simulink model "MHILSimHWImpl"  (R2024a)
settings: Solver=FixedStepDiscrete  StartTime=0.0  StopTime=2e-4  FixedStep=4e-9  RelTol=1e-3
values from neighbouring files (symbols this model uses):
  cfg = tddbl_model    [HILSimModel.m]
undefined symbols (not defined in the file or in its folder): AXI4, dt, hw, ip, Lite, xc7z020clg400
libraries: hdlBasic x1497, hdlUtilities x3, vmcUtilities x1
(part 5 of 11)

== system MHILSimHWImpl/hilsim_ipcore/proc_domain/sel_addrs_slice_2 ==
  Bus Creator : BusCreator  Inputs=6
  Constant : hdlBasic/Constant  const=ip.nlfaddr.slice2_u0  gui_display_data_type=Fixed-point  arith_type=Unsigned  n_bits=8  bin_pt=0  preci_type=Single  exp_width=8  frac_width=24  explicit_period=off  period=1  XmcBlockStatus=1  maskContainerNames=tabcontainer1  block_type=constant  block_config=sysgen:Constant_config
  Constant1 : hdlBasic/Constant  const=ip.nlfaddr.slice2_u1  gui_display_data_type=Fixed-point  arith_type=Unsigned  n_bits=8  bin_pt=0  preci_type=Single  exp_width=8  frac_width=24  explicit_period=off  period=1  XmcBlockStatus=1  maskContainerNames=tabcontainer1  block_type=constant  block_config=sysgen:Constant_config
  Constant2 : hdlBasic/Constant  const=ip.nlfaddr.slice2_x0  gui_display_data_type=Fixed-point  arith_type=Unsigned  n_bits=8  bin_pt=0  preci_type=Single  exp_width=8  frac_width=24  explicit_period=off  period=1  XmcBlockStatus=1  maskContainerNames=tabcontainer1  block_type=constant  block_config=sysgen:Constant_config
  Constant3 : hdlBasic/Constant  const=ip.nlfaddr.slice2_x1  gui_display_data_type=Fixed-point  arith_type=Unsigned  n_bits=8  bin_pt=0  preci_type=Single  exp_width=8  frac_width=24  explicit_period=off  period=1  XmcBlockStatus=1  maskContainerNames=tabcontainer1  block_type=constant  block_config=sysgen:Constant_config
  Constant4 : hdlBasic/Constant  const=ip.nlfaddr.slice2_xd0  gui_display_data_type=Fixed-point  arith_type=Unsigned  n_bits=8  bin_pt=0  preci_type=Single  exp_width=8  frac_width=24  explicit_period=off  period=1  XmcBlockStatus=1  maskContainerNames=tabcontainer1  block_type=constant  block_config=sysgen:Constant_config
  Constant5 : hdlBasic/Constant  const=ip.nlfaddr.slice2_xd1  gui_display_data_type=Fixed-point  arith_type=Unsigned  n_bits=8  bin_pt=0  preci_type=Single  exp_width=8  frac_width=24  explicit_period=off  period=1  XmcBlockStatus=1  maskContainerNames=tabcontainer1  block_type=constant  block_config=sysgen:Constant_config
  nlf_sel_addrs : Outport
  wires:
  Bus Creator/1 -> nlf_sel_addrs/1
  Constant/1 -> Bus Creator/1  "sel_u0"
  Constant1/1 -> Bus Creator/2  "sel_u1"
  Constant2/1 -> Bus Creator/3  "sel_x0"
  Constant3/1 -> Bus Creator/4  "sel_x1"
  Constant4/1 -> Bus Creator/5  "sel_xd0"
  Constant5/1 -> Bus Creator/6  "sel_xd1"

== system MHILSimHWImpl/hilsim_ipcore/proc_domain/slice_0 ==
  note: clk=3
  note: clk=6 (linear)
      | clk=18 (nonlinear)
  note: FB: max_clk=32
  note: clk=3
  note: clk=5
  note: clk=5
  u : Inport
  nlf_cfg_bus : Inport  Port=2
  slice_cfg : Inport  Port=3
  nlf_switch_bus : Inport  Port=4
  nlf_sel_addrs : Inport  Port=5
  reset_in : Inport  Port=6
  Bus Selector : BusSelector  OutputSignals=signal1,signal2,signal3,signal4,signal5,signal6,signal7,signal8,signal9,signal10,signal11,signal12,signal13,signal14,signal15,signal16
  Register{1..10,12} (11 alike) : hdlBasic/Register  init=0  rst=off  en=off  XmcBlockStatus=1  maskContainerNames=tabcontainer1  block_type=register  block_config=sysgen:Register_config
  fb_func : Subsystem
  fb_resync : Subsystem
  int_xddot_xdot : Subsystem
  int_xdot_x : Subsystem
  sample_sync : hdlUtilities/Clock Enable Probe  inherit_constraints=on  XmcBlockStatus=1  maskContainerNames=group1  block_type=ceprobe  block_config=sysgen:CEProbe_config
  u_downsample : hdlBasic/Down Sample  sample_ratio=hw.oversample  sample_phase=First Value of Frame  en=off  rst=off  latency=0  XmcBlockStatus=1  maskContainerNames=group1  block_type=dsamp  block_config=sysgen:Downsample_config
  u_upsample : hdlBasic/Up Sample  sample_ratio=hw.oversample  copy_samples=on  en=off  latency=1  XmcBlockStatus=1  maskContainerNames=group1  block_type=usamp  block_config=sysgen:Upsample_config
  x_psc : Subsystem
  xdot_psc : Subsystem
  x_sync : Outport
  xd_sync : Outport  Port=2
  xdd_sync : Outport  Port=3
  wires:
  x_psc/1(out) -> fb_resync/4(x)
  xdot_psc/1(out) -> fb_resync/5(xd), int_xdot_x/3(xdot)
  fb_func/1(xdd) -> int_xddot_xdot/3(xdot), fb_resync/6(xdd)
  sample_sync/1 -> fb_resync/1(ts_sync_in), int_xddot_xdot/1(ts_sync_in), int_xdot_x/1(ts_sync_in)
  nlf_cfg_bus/1 -> fb_func/4(nlf_cfg_bus)
  int_xdot_x/1(x) -> x_psc/1(in)
  u_downsample/1 -> sample_sync/1, u_upsample/1
  fb_resync/1(u_sync) -> fb_func/1(u)
  Bus Selector/1 -> fb_func/7(x_mux)  "<signal1>"
  Bus Selector/2 -> Register4/1  "<signal2>"
  Bus Selector/3 -> fb_func/9(x_nlf_presc)  "<signal3>"
  Bus Selector/4 -> fb_func/10(x_nlf_gain)  "<signal4>"
  Bus Selector/5 -> fb_func/11(xd_mux)  "<signal5>"
  Bus Selector/6 -> Register5/1  "<signal6>"
  Bus Selector/7 -> fb_func/13(xd_nlf_presc)  "<signal7>"
  Bus Selector/8 -> fb_func/14(xd_nlf_gain)  "<signal8>"
  Bus Selector/9 -> fb_func/15(u_mux)  "<signal9>"
  Bus Selector/10 -> Register6/1  "<signal10>"
  Bus Selector/11 -> fb_func/17(u_nlf_presc)  "<signal11>"
  Bus Selector/12 -> fb_func/18(u_nlf_gain)  "<signal12>"
  slice_cfg/1 -> Bus Selector/1
  int_xddot_xdot/1(x) -> xdot_psc/1(in)
  Bus Selector/13 -> Register12/1  "<signal13>"
  Bus Selector/14 -> Register1/1  "<signal14>"
  Bus Selector/15 -> Register2/1  "<signal15>"
  Bus Selector/16 -> Register3/1  "<signal16>"
  u_upsample/1 -> fb_resync/3(u)
  fb_resync/2(x_sync) -> x_sync/1, fb_func/2(x)
  fb_resync/3(xd_sync) -> xd_sync/1, fb_func/3(xd)
  u/1 -> u_downsample/1
  Register12/1 -> Register8/1
  Register1/1 -> Register7/1
  Register2/1 -> Register9/1
  Register3/1 -> Register10/1
  Register4/1 -> fb_func/8(x_gain)
  Register5/1 -> fb_func/12(xd_gain)
  Register6/1 -> fb_func/16(u_gain)
  reset_in/1 -> fb_resync/2(reset_in), int_xdot_x/2(reset_in), int_xddot_xdot/2(reset_in)
  Register8/1 -> xdot_psc/2(presc_shift)
  Register7/1 -> xdot_psc/3(presc_mul)
  Register10/1 -> x_psc/3(presc_mul)
  Register9/1 -> x_psc/2(presc_shift)
  fb_resync/4(xdd_sync) -> xdd_sync/1
  nlf_switch_bus/1 -> fb_func/5(nlf_switch_bus)
  nlf_sel_addrs/1 -> fb_func/6(nlf_sel_addrs)

== system MHILSimHWImpl/hilsim_ipcore/proc_domain/slice_1 ==
  note: clk=3
  note: clk=6 (linear)
      | clk=18 (nonlinear)
  note: FB: max_clk=32
  note: clk=3
  note: clk=5
  note: clk=5
  u : Inport
  nlf_cfg_bus : Inport  Port=2
  slice_cfg : Inport  Port=3
  nlf_switch_bus : Inport  Port=4
  nlf_sel_addrs : Inport  Port=5
  reset_in : Inport  Port=6
  Bus Selector : BusSelector  OutputSignals=signal1,signal2,signal3,signal4,signal5,signal6,signal7,signal8,signal9,signal10,signal11,signal12,signal13,signal14,signal15,signal16
  Register{1..10,12} (11 alike) : hdlBasic/Register  init=0  rst=off  en=off  XmcBlockStatus=1  maskContainerNames=tabcontainer1  block_type=register  block_config=sysgen:Register_config
  fb_func : Subsystem
  fb_resync : Subsystem
  int_xddot_xdot : Subsystem
  int_xdot_x : Subsystem
  sample_sync : hdlUtilities/Clock Enable Probe  inherit_constraints=on  XmcBlockStatus=1  maskContainerNames=group1  block_type=ceprobe  block_config=sysgen:CEProbe_config
  u_downsample : hdlBasic/Down Sample  sample_ratio=hw.oversample  sample_phase=First Value of Frame  en=off  rst=off  latency=0  XmcBlockStatus=1  maskContainerNames=group1  block_type=dsamp  block_config=sysgen:Downsample_config
  u_upsample : hdlBasic/Up Sample  sample_ratio=hw.oversample  copy_samples=on  en=off  latency=1  XmcBlockStatus=1  maskContainerNames=group1  block_type=usamp  block_config=sysgen:Upsample_config
  x_psc : Subsystem
  xdot_psc : Subsystem
  x_sync : Outport
  xd_sync : Outport  Port=2
  xdd_sync : Outport  Port=3
  wires:
  x_psc/1(out) -> fb_resync/4(x)
  xdot_psc/1(out) -> fb_resync/5(xd), int_xdot_x/3(xdot)
  fb_func/1(xdd) -> int_xddot_xdot/3(xdot), fb_resync/6(xdd)
  sample_sync/1 -> fb_resync/1(ts_sync_in), int_xddot_xdot/1(ts_sync_in), int_xdot_x/1(ts_sync_in)
  nlf_cfg_bus/1 -> fb_func/4(nlf_cfg_bus)
  int_xdot_x/1(x) -> x_psc/1(in)
  u_downsample/1 -> sample_sync/1, u_upsample/1
  fb_resync/1(u_sync) -> fb_func/1(u)
  Bus Selector/1 -> fb_func/7(x_mux)  "<signal1>"
  Bus Selector/2 -> Register4/1  "<signal2>"
  Bus Selector/3 -> fb_func/9(x_nlf_presc)  "<signal3>"
  Bus Selector/4 -> fb_func/10(x_nlf_gain)  "<signal4>"
  Bus Selector/5 -> fb_func/11(xd_mux)  "<signal5>"
  Bus Selector/6 -> Register5/1  "<signal6>"
  Bus Selector/7 -> fb_func/13(xd_nlf_presc)  "<signal7>"
  Bus Selector/8 -> fb_func/14(xd_nlf_gain)  "<signal8>"
  Bus Selector/9 -> fb_func/15(u_mux)  "<signal9>"
  Bus Selector/10 -> Register6/1  "<signal10>"
  Bus Selector/11 -> fb_func/17(u_nlf_presc)  "<signal11>"
  Bus Selector/12 -> fb_func/18(u_nlf_gain)  "<signal12>"
  slice_cfg/1 -> Bus Selector/1
  int_xddot_xdot/1(x) -> xdot_psc/1(in)
  Bus Selector/13 -> Register12/1  "<signal13>"
  Bus Selector/14 -> Register1/1  "<signal14>"
  Bus Selector/15 -> Register2/1  "<signal15>"
  Bus Selector/16 -> Register3/1  "<signal16>"
  u_upsample/1 -> fb_resync/3(u)
  fb_resync/2(x_sync) -> x_sync/1, fb_func/2(x)
  fb_resync/3(xd_sync) -> xd_sync/1, fb_func/3(xd)
  u/1 -> u_downsample/1
  Register12/1 -> Register8/1
  Register1/1 -> Register7/1
  Register2/1 -> Register9/1
  Register3/1 -> Register10/1
  Register4/1 -> fb_func/8(x_gain)
  Register5/1 -> fb_func/12(xd_gain)
  Register6/1 -> fb_func/16(u_gain)
  reset_in/1 -> fb_resync/2(reset_in), int_xdot_x/2(reset_in), int_xddot_xdot/2(reset_in)
  Register8/1 -> xdot_psc/2(presc_shift)
  Register7/1 -> xdot_psc/3(presc_mul)
  Register10/1 -> x_psc/3(presc_mul)
  Register9/1 -> x_psc/2(presc_shift)
  fb_resync/4(xdd_sync) -> xdd_sync/1
  nlf_switch_bus/1 -> fb_func/5(nlf_switch_bus)
  nlf_sel_addrs/1 -> fb_func/6(nlf_sel_addrs)

== system MHILSimHWImpl/hilsim_ipcore/proc_domain/slice_2 ==
  note: clk=3
  note: clk=6 (linear)
      | clk=18 (nonlinear)
  note: FB: max_clk=32
  note: clk=3
  note: clk=5
  note: clk=5
  u : Inport
  nlf_cfg_bus : Inport  Port=2
  slice_cfg : Inport  Port=3
  nlf_switch_bus : Inport  Port=4
  nlf_sel_addrs : Inport  Port=5
  reset_in : Inport  Port=6
  Bus Selector : BusSelector  OutputSignals=signal1,signal2,signal3,signal4,signal5,signal6,signal7,signal8,signal9,signal10,signal11,signal12,signal13,signal14,signal15,signal16
  Register{1..10,12} (11 alike) : hdlBasic/Register  init=0  rst=off  en=off  XmcBlockStatus=1  maskContainerNames=tabcontainer1  block_type=register  block_config=sysgen:Register_config
  fb_func : Subsystem
  fb_resync : Subsystem
  int_xddot_xdot : Subsystem
  int_xdot_x : Subsystem
  sample_sync : hdlUtilities/Clock Enable Probe  inherit_constraints=on  XmcBlockStatus=1  maskContainerNames=group1  block_type=ceprobe  block_config=sysgen:CEProbe_config
  u_downsample : hdlBasic/Down Sample  sample_ratio=hw.oversample  sample_phase=First Value of Frame  en=off  rst=off  latency=0  XmcBlockStatus=1  maskContainerNames=group1  block_type=dsamp  block_config=sysgen:Downsample_config
  u_upsample : hdlBasic/Up Sample  sample_ratio=hw.oversample  copy_samples=on  en=off  latency=1  XmcBlockStatus=1  maskContainerNames=group1  block_type=usamp  block_config=sysgen:Upsample_config
  x_psc : Subsystem
  xdot_psc : Subsystem
  x_sync : Outport
  xd_sync : Outport  Port=2
  xdd_sync : Outport  Port=3
  wires:
  x_psc/1(out) -> fb_resync/4(x)
  xdot_psc/1(out) -> fb_resync/5(xd), int_xdot_x/3(xdot)
  fb_func/1(xdd) -> int_xddot_xdot/3(xdot), fb_resync/6(xdd)
  sample_sync/1 -> fb_resync/1(ts_sync_in), int_xddot_xdot/1(ts_sync_in), int_xdot_x/1(ts_sync_in)
  nlf_cfg_bus/1 -> fb_func/4(nlf_cfg_bus)
  int_xdot_x/1(x) -> x_psc/1(in)
  u_downsample/1 -> sample_sync/1, u_upsample/1
  fb_resync/1(u_sync) -> fb_func/1(u)
  Bus Selector/1 -> fb_func/7(x_mux)  "<signal1>"
  Bus Selector/2 -> Register4/1  "<signal2>"
  Bus Selector/3 -> fb_func/9(x_nlf_presc)  "<signal3>"
  Bus Selector/4 -> fb_func/10(x_nlf_gain)  "<signal4>"
  Bus Selector/5 -> fb_func/11(xd_mux)  "<signal5>"
  Bus Selector/6 -> Register5/1  "<signal6>"
  Bus Selector/7 -> fb_func/13(xd_nlf_presc)  "<signal7>"
  Bus Selector/8 -> fb_func/14(xd_nlf_gain)  "<signal8>"
  Bus Selector/9 -> fb_func/15(u_mux)  "<signal9>"
  Bus Selector/10 -> Register6/1  "<signal10>"
  Bus Selector/11 -> fb_func/17(u_nlf_presc)  "<signal11>"
  Bus Selector/12 -> fb_func/18(u_nlf_gain)  "<signal12>"
  slice_cfg/1 -> Bus Selector/1
  int_xddot_xdot/1(x) -> xdot_psc/1(in)
  Bus Selector/13 -> Register12/1  "<signal13>"
  Bus Selector/14 -> Register1/1  "<signal14>"
  Bus Selector/15 -> Register2/1  "<signal15>"
  Bus Selector/16 -> Register3/1  "<signal16>"
  u_upsample/1 -> fb_resync/3(u)
  fb_resync/2(x_sync) -> x_sync/1, fb_func/2(x)
  fb_resync/3(xd_sync) -> xd_sync/1, fb_func/3(xd)
  u/1 -> u_downsample/1
  Register12/1 -> Register8/1
  Register1/1 -> Register7/1
  Register2/1 -> Register9/1
  Register3/1 -> Register10/1
  Register4/1 -> fb_func/8(x_gain)
  Register5/1 -> fb_func/12(xd_gain)
  Register6/1 -> fb_func/16(u_gain)
  reset_in/1 -> fb_resync/2(reset_in), int_xdot_x/2(reset_in), int_xddot_xdot/2(reset_in)
  Register8/1 -> xdot_psc/2(presc_shift)
  Register7/1 -> xdot_psc/3(presc_mul)
  Register10/1 -> x_psc/3(presc_mul)
  Register9/1 -> x_psc/2(presc_shift)
  fb_resync/4(xdd_sync) -> xdd_sync/1
  nlf_switch_bus/1 -> fb_func/5(nlf_switch_bus)
  nlf_sel_addrs/1 -> fb_func/6(nlf_sel_addrs)

== system MHILSimHWImpl/hilsim_ipcore/proc_domain/adc_nlf/nlf_adc0 ==
  note: Signal should now be normalized
      | to range -1 to 1.
  x : Inport
  presc : Inport  Port=2
  gain : Inport  Port=3
  cfg_select : Inport  Port=4
  cfg_addr : Inport  Port=5
  cfg_data : Inport  Port=6
  cfg_we : Inport  Port=7
  AddSub : hdlBasic/AddSub  mode=Addition  use_carryin=off  use_carryout=off  en=off  latency=1  precision=User Defined  arith_type=Unsigned  n_bits=ip.f_nlf.lut_addr_bits  bin_pt=0  quantization=Truncate  overflow=Wrap  use_behavioral_HDL=off  hw_selection=Fabric  pipelined=off  XmcBlockStatus=1  maskContainerNames=tabcontainer1  block_type=addsub  block_config=sysgen:Addsub_config
  AddSub1 : hdlBasic/AddSub  mode=Subtraction  use_carryin=off  use_carryout=off  en=off  latency=2  precision=User Defined  arith_type="Signed  (2's comp)"  n_bits=dt.slice.sz  bin_pt=dt.slice.bin  quantization=Truncate  overflow=Wrap  use_behavioral_HDL=off  hw_selection=Fabric  pipelined=off  XmcBlockStatus=1  maskContainerNames=tabcontainer1  block_type=addsub  block_config=sysgen:Addsub_config
  LUT : hdlBasic/Dual Port RAM  depth=ip.f_nlf.lut_sz  initVector=cfg.adc0_nlf.lut  distributed_mem=Block RAM  init_a=0  init_b=0  rst_a=off  rst_b=off  en_a=off  en_b=off  latency=1  write_mode_A=Read After Write  write_mode_B=Read After Write  explicit_period=[]  period=[]  simulation_type=fast_sim  XmcBlockStatus=1  maskContainerNames=tabcontainer1  block_type=dpram  block_config=sysgen:Dpram_config  optimize=Area
      settings: infoedit=[]
  Reinterpret : hdlBasic/Reinterpret  force_arith_type=on  arith_type=Unsigned  force_bin_pt=on  bin_pt=0  XmcBlockStatus=1  maskContainerNames=group1  block_type=reinterpret  block_config=sysgen:Reinterpret_config
  add_interpolate : hdlBasic/AddSub  mode=Addition  use_carryin=off  use_carryout=off  en=off  latency=1  precision=User Defined  arith_type="Signed  (2's comp)"  n_bits=dt.slice.sz  bin_pt=dt.slice.bin  quantization=Truncate  overflow=Wrap  use_behavioral_HDL=off  hw_selection=Fabric  pipelined=off  XmcBlockStatus=1  maskContainerNames=tabcontainer1  block_type=addsub  block_config=sysgen:Addsub_config
  addra_mux : hdlBasic/Mux  inputs=2  en=off  latency=1  precision=Full  arith_type=Unsigned  n_bits=16  bin_pt=14  quantization=Truncate  overflow=Wrap  XmcBlockStatus=1  maskContainerNames=tabcontainer1  block_type=mux  block_config=sysgen:Mux_config
  bool_zero_we : hdlBasic/Constant  const=0  gui_display_data_type=Boolean  arith_type=Boolean  n_bits=16  bin_pt=14  preci_type=Single  exp_width=8  frac_width=24  explicit_period=off  period=1  XmcBlockStatus=1  maskContainerNames=tabcontainer1  block_type=constant  block_config=sysgen:Constant_config
  bool_zero_wea : hdlBasic/Constant  const=0  gui_display_data_type=Boolean  arith_type=Boolean  n_bits=16  bin_pt=14  preci_type=Single  exp_width=8  frac_width=24  explicit_period=off  period=1  XmcBlockStatus=1  maskContainerNames=tabcontainer1  block_type=constant  block_config=sysgen:Constant_config
  cast_cutoff_lsbits : hdlBasic/Convert  gui_display_data_type=Fixed-point  arith_type="Signed  (2's comp)"  n_bits=ip.f_nlf.lut_addr_bits  bin_pt=ip.f_nlf.lut_addr_bits-1  float_type=Single  exp_bits=8  fraction_bits=24  quantization=Truncate  overflow=Wrap  en=off  latency=0  pipeline=off  XmcBlockStatus=1  maskContainerNames=group2  block_type=convert  block_config=sysgen:Convert_config  block_width=595  block_height=885
  cast_to_dt/slice : hdlBasic/Convert  gui_display_data_type=Fixed-point  arith_type="Signed  (2's comp)"  n_bits=dt.slice.sz  bin_pt=dt.slice.bin  float_type=Single  exp_bits=8  fraction_bits=24  quantization=Truncate  overflow=Wrap  en=off  latency=0  pipeline=off  XmcBlockStatus=1  maskContainerNames=group2  block_type=convert  block_config=sysgen:Convert_config  block_width=595  block_height=885
  const_1 : hdlBasic/Constant  const=1.0  gui_display_data_type=Fixed-point  arith_type=Unsigned  n_bits=ip.f_nlf.lut_addr_bits  bin_pt=0  preci_type=Single  exp_width=8  frac_width=24  explicit_period=off  period=1  XmcBlockStatus=1  maskContainerNames=tabcontainer1  block_type=constant  block_config=sysgen:Constant_config
  const_1_interp : hdlBasic/Constant  const=1  gui_display_data_type=Fixed-point  arith_type=Signed (2's comp)  n_bits=dt.slice.sz  bin_pt=dt.slice.bin  preci_type=Single  exp_width=8  frac_width=24  explicit_period=off  period=1  XmcBlockStatus=1  maskContainerNames=tabcontainer1  block_type=constant  block_config=sysgen:Constant_config
  cutoff_msbits : hdlBasic/Slice  nbits=dt.slice.sz - ip.f_nlf.lut_addr_bits-1  boolean_output=off  mode=Lower Bit Location + Width  bit1=0  base1=MSB of Input  bit0=0  base0=LSB of Input  XmcBlockStatus=1  maskContainerNames=group1  block_type=slice  block_config=sysgen:Slice_config
  delay_sync_interpolate : hdlBasic/Delay  rst=off  en=off  latency=2  reg_retiming=off  XmcBlockStatus=1  maskContainerNames=group1  block_type=delay  block_config=sysgen:Delay_config
  dina_mux : hdlBasic/Mux  inputs=2  en=off  latency=1  precision=Full  arith_type=Unsigned  n_bits=16  bin_pt=14  quantization=Truncate  overflow=Wrap  XmcBlockStatus=1  maskContainerNames=tabcontainer1  block_type=mux  block_config=sysgen:Mux_config
  mult_a : hdlBasic/Mult  precision=User Defined  arith_type="Signed  (2's comp)"  n_bits=dt.slice.sz  bin_pt=dt.slice.bin  quantization=Truncate  overflow=Wrap  en=off  latency=3  opt_float=off  fp_mult_usage=No Usage  use_behavioral_HDL=off  opt=Speed  use_embedded=on  optimum_pipeline=off  pipeline=on  use_rpm=on  placement_style=Triangular  XmcBlockStatus=1  maskContainerNames=group1  block_type=mult  block_config=sysgen:Mult_config  block_width=598  block_height=876
  mult_b : hdlBasic/Mult  precision=User Defined  arith_type="Signed  (2's comp)"  n_bits=dt.slice.sz  bin_pt=dt.slice.bin  quantization=Truncate  overflow=Wrap  en=off  latency=3  opt_float=off  fp_mult_usage=No Usage  use_behavioral_HDL=off  opt=Speed  use_embedded=on  optimum_pipeline=off  pipeline=on  use_rpm=on  placement_style=Triangular  XmcBlockStatus=1  maskContainerNames=group1  block_type=mult  block_config=sysgen:Mult_config  block_width=598  block_height=876
  mult_inp_scale : hdlBasic/Mult  precision=User Defined  arith_type="Signed  (2's comp)"  n_bits=dt.slice.sz  bin_pt=dt.slice.sz - 2  quantization=Truncate  overflow=Wrap  en=off  latency=3  opt_float=off  fp_mult_usage=No Usage  use_behavioral_HDL=off  opt=Speed  use_embedded=on  optimum_pipeline=off  pipeline=on  use_rpm=on  placement_style=Triangular  XmcBlockStatus=1  maskContainerNames=group1  block_type=mult  block_config=sysgen:Mult_config  block_width=598  block_height=876
  mult_out_scale : hdlBasic/Mult  precision=User Defined  arith_type="Signed  (2's comp)"  n_bits=dt.slice.sz  bin_pt=dt.slice.bin  quantization=Truncate  overflow=Wrap  en=off  latency=3  opt_float=off  fp_mult_usage=No Usage  use_behavioral_HDL=off  opt=Speed  use_embedded=on  optimum_pipeline=off  pipeline=on  use_rpm=on  placement_style=Triangular  XmcBlockStatus=1  maskContainerNames=group1  block_type=mult  block_config=sysgen:Mult_config  block_width=598  block_height=876
  reint_sliced : hdlBasic/Reinterpret  force_arith_type=on  arith_type=Unsigned  force_bin_pt=on  bin_pt=dt.slice.sz - ip.f_nlf.lut_addr_bits-1  XmcBlockStatus=1  maskContainerNames=group1  block_type=reinterpret  block_config=sysgen:Reinterpret_config
  wea_mux : hdlBasic/Mux  inputs=2  en=off  latency=1  precision=Full  arith_type=Unsigned  n_bits=16  bin_pt=14  quantization=Truncate  overflow=Wrap  XmcBlockStatus=1  maskContainerNames=tabcontainer1  block_type=mux  block_config=sysgen:Mux_config
  zero_nlf_datatype : hdlBasic/Constant  const=0  gui_display_data_type=Fixed-point  arith_type=Signed (2's comp)  n_bits=dt.nlf.sz  bin_pt=dt.nlf.bin  preci_type=Single  exp_width=8  frac_width=24  explicit_period=off  period=1  XmcBlockStatus=1  maskContainerNames=tabcontainer1  block_type=constant  block_config=sysgen:Constant_config
  zero_nlf_dina : hdlBasic/Constant  const=0  gui_display_data_type=Fixed-point  arith_type=Signed (2's comp)  n_bits=dt.nlf.sz  bin_pt=dt.nlf.bin  preci_type=Single  exp_width=8  frac_width=24  explicit_period=off  period=1  XmcBlockStatus=1  maskContainerNames=tabcontainer1  block_type=constant  block_config=sysgen:Constant_config
  f(x) : Outport
  wires:
  x/1 -> mult_inp_scale/1
  presc/1 -> mult_inp_scale/2
  cast_cutoff_lsbits/1 -> Reinterpret/1
  Reinterpret/1 -> addra_mux/2, AddSub/1
  const_1/1 -> AddSub/2
  AddSub/1 -> LUT/4
  bool_zero_we/1 -> LUT/6
  zero_nlf_datatype/1 -> LUT/5
  LUT/2 -> mult_b/1
  LUT/1 -> mult_a/1
  mult_inp_scale/1 -> cast_cutoff_lsbits/1, cutoff_msbits/1
  cutoff_msbits/1 -> reint_sliced/1
  reint_sliced/1 -> cast_to_dt/slice/1
  cast_to_dt/slice/1 -> AddSub1/2, delay_sync_interpolate/1
  const_1_interp/1 -> AddSub1/1
  delay_sync_interpolate/1 -> mult_b/2
  AddSub1/1 -> mult_a/2
  mult_a/1 -> add_interpolate/1
  mult_b/1 -> add_interpolate/2
  gain/1 -> mult_out_scale/2
  mult_out_scale/1 -> f(x)/1
  dina_mux/1 -> LUT/2
  addra_mux/1 -> LUT/1
  wea_mux/1 -> LUT/3
  bool_zero_wea/1 -> wea_mux/2
  zero_nlf_dina/1 -> dina_mux/2
  cfg_select/1 -> wea_mux/1, dina_mux/1, addra_mux/1
  cfg_addr/1 -> addra_mux/3
  cfg_data/1 -> dina_mux/3
  cfg_we/1 -> wea_mux/3
  add_interpolate/1 -> mult_out_scale/1

== system MHILSimHWImpl/hilsim_ipcore/proc_domain/adc_nlf/nlf_adc1 ==
  note: Signal should now be normalized
      | to range -1 to 1.
  x : Inport
  presc : Inport  Port=2
  gain : Inport  Port=3
  cfg_select : Inport  Port=4
  cfg_addr : Inport  Port=5
  cfg_data : Inport  Port=6
  cfg_we : Inport  Port=7
  AddSub : hdlBasic/AddSub  mode=Addition  use_carryin=off  use_carryout=off  en=off  latency=1  precision=User Defined  arith_type=Unsigned  n_bits=ip.f_nlf.lut_addr_bits  bin_pt=0  quantization=Truncate  overflow=Wrap  use_behavioral_HDL=off  hw_selection=Fabric  pipelined=off  XmcBlockStatus=1  maskContainerNames=tabcontainer1  block_type=addsub  block_config=sysgen:Addsub_config
  AddSub1 : hdlBasic/AddSub  mode=Subtraction  use_carryin=off  use_carryout=off  en=off  latency=2  precision=User Defined  arith_type="Signed  (2's comp)"  n_bits=dt.slice.sz  bin_pt=dt.slice.bin  quantization=Truncate  overflow=Wrap  use_behavioral_HDL=off  hw_selection=Fabric  pipelined=off  XmcBlockStatus=1  maskContainerNames=tabcontainer1  block_type=addsub  block_config=sysgen:Addsub_config
  LUT : hdlBasic/Dual Port RAM  depth=ip.f_nlf.lut_sz  initVector=cfg.adc1_nlf.lut  distributed_mem=Block RAM  init_a=0  init_b=0  rst_a=off  rst_b=off  en_a=off  en_b=off  latency=1  write_mode_A=Read After Write  write_mode_B=Read After Write  explicit_period=[]  period=[]  simulation_type=fast_sim  XmcBlockStatus=1  maskContainerNames=tabcontainer1  block_type=dpram  block_config=sysgen:Dpram_config  optimize=Area
      settings: infoedit=[]
  Reinterpret : hdlBasic/Reinterpret  force_arith_type=on  arith_type=Unsigned  force_bin_pt=on  bin_pt=0  XmcBlockStatus=1  maskContainerNames=group1  block_type=reinterpret  block_config=sysgen:Reinterpret_config
  add_interpolate : hdlBasic/AddSub  mode=Addition  use_carryin=off  use_carryout=off  en=off  latency=1  precision=User Defined  arith_type="Signed  (2's comp)"  n_bits=dt.slice.sz  bin_pt=dt.slice.bin  quantization=Truncate  overflow=Wrap  use_behavioral_HDL=off  hw_selection=Fabric  pipelined=off  XmcBlockStatus=1  maskContainerNames=tabcontainer1  block_type=addsub  block_config=sysgen:Addsub_config
  addra_mux : hdlBasic/Mux  inputs=2  en=off  latency=1  precision=Full  arith_type=Unsigned  n_bits=16  bin_pt=14  quantization=Truncate  overflow=Wrap  XmcBlockStatus=1  maskContainerNames=tabcontainer1  block_type=mux  block_config=sysgen:Mux_config
  bool_zero_we : hdlBasic/Constant  const=0  gui_display_data_type=Boolean  arith_type=Boolean  n_bits=16  bin_pt=14  preci_type=Single  exp_width=8  frac_width=24  explicit_period=off  period=1  XmcBlockStatus=1  maskContainerNames=tabcontainer1  block_type=constant  block_config=sysgen:Constant_config
  bool_zero_wea : hdlBasic/Constant  const=0  gui_display_data_type=Boolean  arith_type=Boolean  n_bits=16  bin_pt=14  preci_type=Single  exp_width=8  frac_width=24  explicit_period=off  period=1  XmcBlockStatus=1  maskContainerNames=tabcontainer1  block_type=constant  block_config=sysgen:Constant_config
  cast_cutoff_lsbits : hdlBasic/Convert  gui_display_data_type=Fixed-point  arith_type="Signed  (2's comp)"  n_bits=ip.f_nlf.lut_addr_bits  bin_pt=ip.f_nlf.lut_addr_bits-1  float_type=Single  exp_bits=8  fraction_bits=24  quantization=Truncate  overflow=Wrap  en=off  latency=0  pipeline=off  XmcBlockStatus=1  maskContainerNames=group2  block_type=convert  block_config=sysgen:Convert_config  block_width=595  block_height=885
  cast_to_dt/slice : hdlBasic/Convert  gui_display_data_type=Fixed-point  arith_type="Signed  (2's comp)"  n_bits=dt.slice.sz  bin_pt=dt.slice.bin  float_type=Single  exp_bits=8  fraction_bits=24  quantization=Truncate  overflow=Wrap  en=off  latency=0  pipeline=off  XmcBlockStatus=1  maskContainerNames=group2  block_type=convert  block_config=sysgen:Convert_config  block_width=595  block_height=885
  const_1 : hdlBasic/Constant  const=1.0  gui_display_data_type=Fixed-point  arith_type=Unsigned  n_bits=ip.f_nlf.lut_addr_bits  bin_pt=0  preci_type=Single  exp_width=8  frac_width=24  explicit_period=off  period=1  XmcBlockStatus=1  maskContainerNames=tabcontainer1  block_type=constant  block_config=sysgen:Constant_config
  const_1_interp : hdlBasic/Constant  const=1  gui_display_data_type=Fixed-point  arith_type=Signed (2's comp)  n_bits=dt.slice.sz  bin_pt=dt.slice.bin  preci_type=Single  exp_width=8  frac_width=24  explicit_period=off  period=1  XmcBlockStatus=1  maskContainerNames=tabcontainer1  block_type=constant  block_config=sysgen:Constant_config
  cutoff_msbits : hdlBasic/Slice  nbits=dt.slice.sz - ip.f_nlf.lut_addr_bits-1  boolean_output=off  mode=Lower Bit Location + Width  bit1=0  base1=MSB of Input  bit0=0  base0=LSB of Input  XmcBlockStatus=1  maskContainerNames=group1  block_type=slice  block_config=sysgen:Slice_config
  delay_sync_interpolate : hdlBasic/Delay  rst=off  en=off  latency=2  reg_retiming=off  XmcBlockStatus=1  maskContainerNames=group1  block_type=delay  block_config=sysgen:Delay_config
  dina_mux : hdlBasic/Mux  inputs=2  en=off  latency=1  precision=Full  arith_type=Unsigned  n_bits=16  bin_pt=14  quantization=Truncate  overflow=Wrap  XmcBlockStatus=1  maskContainerNames=tabcontainer1  block_type=mux  block_config=sysgen:Mux_config
  mult_a : hdlBasic/Mult  precision=User Defined  arith_type="Signed  (2's comp)"  n_bits=dt.slice.sz  bin_pt=dt.slice.bin  quantization=Truncate  overflow=Wrap  en=off  latency=3  opt_float=off  fp_mult_usage=No Usage  use_behavioral_HDL=off  opt=Speed  use_embedded=on  optimum_pipeline=off  pipeline=on  use_rpm=on  placement_style=Triangular  XmcBlockStatus=1  maskContainerNames=group1  block_type=mult  block_config=sysgen:Mult_config  block_width=598  block_height=876
  mult_b : hdlBasic/Mult  precision=User Defined  arith_type="Signed  (2's comp)"  n_bits=dt.slice.sz  bin_pt=dt.slice.bin  quantization=Truncate  overflow=Wrap  en=off  latency=3  opt_float=off  fp_mult_usage=No Usage  use_behavioral_HDL=off  opt=Speed  use_embedded=on  optimum_pipeline=off  pipeline=on  use_rpm=on  placement_style=Triangular  XmcBlockStatus=1  maskContainerNames=group1  block_type=mult  block_config=sysgen:Mult_config  block_width=598  block_height=876
  mult_inp_scale : hdlBasic/Mult  precision=User Defined  arith_type="Signed  (2's comp)"  n_bits=dt.slice.sz  bin_pt=dt.slice.sz - 2  quantization=Truncate  overflow=Wrap  en=off  latency=3  opt_float=off  fp_mult_usage=No Usage  use_behavioral_HDL=off  opt=Speed  use_embedded=on  optimum_pipeline=off  pipeline=on  use_rpm=on  placement_style=Triangular  XmcBlockStatus=1  maskContainerNames=group1  block_type=mult  block_config=sysgen:Mult_config  block_width=598  block_height=876
  mult_out_scale : hdlBasic/Mult  precision=User Defined  arith_type="Signed  (2's comp)"  n_bits=dt.slice.sz  bin_pt=dt.slice.bin  quantization=Truncate  overflow=Wrap  en=off  latency=3  opt_float=off  fp_mult_usage=No Usage  use_behavioral_HDL=off  opt=Speed  use_embedded=on  optimum_pipeline=off  pipeline=on  use_rpm=on  placement_style=Triangular  XmcBlockStatus=1  maskContainerNames=group1  block_type=mult  block_config=sysgen:Mult_config  block_width=598  block_height=876
  reint_sliced : hdlBasic/Reinterpret  force_arith_type=on  arith_type=Unsigned  force_bin_pt=on  bin_pt=dt.slice.sz - ip.f_nlf.lut_addr_bits-1  XmcBlockStatus=1  maskContainerNames=group1  block_type=reinterpret  block_config=sysgen:Reinterpret_config
  wea_mux : hdlBasic/Mux  inputs=2  en=off  latency=1  precision=Full  arith_type=Unsigned  n_bits=16  bin_pt=14  quantization=Truncate  overflow=Wrap  XmcBlockStatus=1  maskContainerNames=tabcontainer1  block_type=mux  block_config=sysgen:Mux_config
  zero_nlf_datatype : hdlBasic/Constant  const=0  gui_display_data_type=Fixed-point  arith_type=Signed (2's comp)  n_bits=dt.nlf.sz  bin_pt=dt.nlf.bin  preci_type=Single  exp_width=8  frac_width=24  explicit_period=off  period=1  XmcBlockStatus=1  maskContainerNames=tabcontainer1  block_type=constant  block_config=sysgen:Constant_config
  zero_nlf_dina : hdlBasic/Constant  const=0  gui_display_data_type=Fixed-point  arith_type=Signed (2's comp)  n_bits=dt.nlf.sz  bin_pt=dt.nlf.bin  preci_type=Single  exp_width=8  frac_width=24  explicit_period=off  period=1  XmcBlockStatus=1  maskContainerNames=tabcontainer1  block_type=constant  block_config=sysgen:Constant_config
  f(x) : Outport
  wires:
  x/1 -> mult_inp_scale/1
  presc/1 -> mult_inp_scale/2
  cast_cutoff_lsbits/1 -> Reinterpret/1
  Reinterpret/1 -> addra_mux/2, AddSub/1
  const_1/1 -> AddSub/2
  AddSub/1 -> LUT/4
  bool_zero_we/1 -> LUT/6
  zero_nlf_datatype/1 -> LUT/5
  LUT/2 -> mult_b/1
  LUT/1 -> mult_a/1
  mult_inp_scale/1 -> cast_cutoff_lsbits/1, cutoff_msbits/1
  cutoff_msbits/1 -> reint_sliced/1
  reint_sliced/1 -> cast_to_dt/slice/1
  cast_to_dt/slice/1 -> AddSub1/2, delay_sync_interpolate/1
  const_1_interp/1 -> AddSub1/1
  delay_sync_interpolate/1 -> mult_b/2
  AddSub1/1 -> mult_a/2
  mult_a/1 -> add_interpolate/1
  mult_b/1 -> add_interpolate/2
  gain/1 -> mult_out_scale/2
  mult_out_scale/1 -> f(x)/1
  dina_mux/1 -> LUT/2
  addra_mux/1 -> LUT/1
  wea_mux/1 -> LUT/3
  bool_zero_wea/1 -> wea_mux/2
  zero_nlf_dina/1 -> dina_mux/2
  cfg_select/1 -> wea_mux/1, dina_mux/1, addra_mux/1
  cfg_addr/1 -> addra_mux/3
  cfg_data/1 -> dina_mux/3
  cfg_we/1 -> wea_mux/3
  add_interpolate/1 -> mult_out_scale/1

== system MHILSimHWImpl/hilsim_ipcore/proc_domain/dac_nlf/nlf_dac0 ==
  note: Signal should now be normalized
      | to range -1 to 1.
  x : Inport
  presc : Inport  Port=2
  gain : Inport  Port=3
  cfg_select : Inport  Port=4
  cfg_addr : Inport  Port=5
  cfg_data : Inport  Port=6
  cfg_we : Inport  Port=7
  AddSub : hdlBasic/AddSub  mode=Addition  use_carryin=off  use_carryout=off  en=off  latency=1  precision=User Defined  arith_type=Unsigned  n_bits=ip.f_nlf.lut_addr_bits  bin_pt=0  quantization=Truncate  overflow=Wrap  use_behavioral_HDL=off  hw_selection=Fabric  pipelined=off  XmcBlockStatus=1  maskContainerNames=tabcontainer1  block_type=addsub  block_config=sysgen:Addsub_config
  AddSub1 : hdlBasic/AddSub  mode=Subtraction  use_carryin=off  use_carryout=off  en=off  latency=2  precision=User Defined  arith_type="Signed  (2's comp)"  n_bits=dt.slice.sz  bin_pt=dt.slice.bin  quantization=Truncate  overflow=Wrap  use_behavioral_HDL=off  hw_selection=Fabric  pipelined=off  XmcBlockStatus=1  maskContainerNames=tabcontainer1  block_type=addsub  block_config=sysgen:Addsub_config
  LUT : hdlBasic/Dual Port RAM  depth=ip.f_nlf.lut_sz  initVector=cfg.dac0_nlf.lut  distributed_mem=Block RAM  init_a=0  init_b=0  rst_a=off  rst_b=off  en_a=off  en_b=off  latency=1  write_mode_A=Read After Write  write_mode_B=Read After Write  explicit_period=[]  period=[]  simulation_type=fast_sim  XmcBlockStatus=1  maskContainerNames=tabcontainer1  block_type=dpram  block_config=sysgen:Dpram_config  optimize=Area
      settings: infoedit=[]
  Reinterpret : hdlBasic/Reinterpret  force_arith_type=on  arith_type=Unsigned  force_bin_pt=on  bin_pt=0  XmcBlockStatus=1  maskContainerNames=group1  block_type=reinterpret  block_config=sysgen:Reinterpret_config
  add_interpolate : hdlBasic/AddSub  mode=Addition  use_carryin=off  use_carryout=off  en=off  latency=1  precision=User Defined  arith_type="Signed  (2's comp)"  n_bits=dt.slice.sz  bin_pt=dt.slice.bin  quantization=Truncate  overflow=Wrap  use_behavioral_HDL=off  hw_selection=Fabric  pipelined=off  XmcBlockStatus=1  maskContainerNames=tabcontainer1  block_type=addsub  block_config=sysgen:Addsub_config
  addra_mux : hdlBasic/Mux  inputs=2  en=off  latency=1  precision=Full  arith_type=Unsigned  n_bits=16  bin_pt=14  quantization=Truncate  overflow=Wrap  XmcBlockStatus=1  maskContainerNames=tabcontainer1  block_type=mux  block_config=sysgen:Mux_config
  bool_zero_we : hdlBasic/Constant  const=0  gui_display_data_type=Boolean  arith_type=Boolean  n_bits=16  bin_pt=14  preci_type=Single  exp_width=8  frac_width=24  explicit_period=off  period=1  XmcBlockStatus=1  maskContainerNames=tabcontainer1  block_type=constant  block_config=sysgen:Constant_config
  bool_zero_wea : hdlBasic/Constant  const=0  gui_display_data_type=Boolean  arith_type=Boolean  n_bits=16  bin_pt=14  preci_type=Single  exp_width=8  frac_width=24  explicit_period=off  period=1  XmcBlockStatus=1  maskContainerNames=tabcontainer1  block_type=constant  block_config=sysgen:Constant_config
  cast_cutoff_lsbits : hdlBasic/Convert  gui_display_data_type=Fixed-point  arith_type=Signed (2's comp)  n_bits=ip.f_nlf.lut_addr_bits  bin_pt=ip.f_nlf.lut_addr_bits-1  float_type=Single  exp_bits=8  fraction_bits=24  quantization=Truncate  overflow=Wrap  en=off  latency=0  pipeline=off  XmcBlockStatus=1  maskContainerNames=group2  block_type=convert  block_config=sysgen:Convert_config  block_width=595  block_height=885
  cast_to_dt/slice : hdlBasic/Convert  gui_display_data_type=Fixed-point  arith_type=Signed (2's comp)  n_bits=dt.slice.sz  bin_pt=dt.slice.bin  float_type=Single  exp_bits=8  fraction_bits=24  quantization=Truncate  overflow=Wrap  en=off  latency=0  pipeline=off  XmcBlockStatus=1  maskContainerNames=group2  block_type=convert  block_config=sysgen:Convert_config  block_width=595  block_height=885
  const_1 : hdlBasic/Constant  const=1.0  gui_display_data_type=Fixed-point  arith_type=Unsigned  n_bits=ip.f_nlf.lut_addr_bits  bin_pt=0  preci_type=Single  exp_width=8  frac_width=24  explicit_period=off  period=1  XmcBlockStatus=1  maskContainerNames=tabcontainer1  block_type=constant  block_config=sysgen:Constant_config
  const_1_interp : hdlBasic/Constant  const=1  gui_display_data_type=Fixed-point  arith_type=Signed (2's comp)  n_bits=dt.slice.sz  bin_pt=dt.slice.bin  preci_type=Single  exp_width=8  frac_width=24  explicit_period=off  period=1  XmcBlockStatus=1  maskContainerNames=tabcontainer1  block_type=constant  block_config=sysgen:Constant_config
  cutoff_msbits : hdlBasic/Slice  nbits=dt.slice.bin - ip.f_nlf.lut_addr_bits + 1  boolean_output=off  mode=Lower Bit Location + Width  bit1=0  base1=MSB of Input  bit0=0  base0=LSB of Input  XmcBlockStatus=1  maskContainerNames=group1  block_type=slice  block_config=sysgen:Slice_config
  delay_sync_interpolate : hdlBasic/Delay  rst=off  en=off  latency=2  reg_retiming=off  XmcBlockStatus=1  maskContainerNames=group1  block_type=delay  block_config=sysgen:Delay_config
  dina_mux : hdlBasic/Mux  inputs=2  en=off  latency=1  precision=Full  arith_type=Unsigned  n_bits=16  bin_pt=14  quantization=Truncate  overflow=Wrap  XmcBlockStatus=1  maskContainerNames=tabcontainer1  block_type=mux  block_config=sysgen:Mux_config
  mult_a : hdlBasic/Mult  precision=User Defined  arith_type="Signed  (2's comp)"  n_bits=dt.slice.sz  bin_pt=dt.slice.bin  quantization=Truncate  overflow=Wrap  en=off  latency=3  use_behavioral_HDL=off  opt=Speed  use_embedded=on  optimum_pipeline=off  pipeline=on  use_rpm=on  placement_style=Triangular  XmcBlockStatus=1  maskContainerNames=group1  block_type=mult  block_config=sysgen:Mult_config  block_width=598  block_height=876
  mult_b : hdlBasic/Mult  precision=User Defined  arith_type="Signed  (2's comp)"  n_bits=dt.slice.sz  bin_pt=dt.slice.bin  quantization=Truncate  overflow=Wrap  en=off  latency=3  use_behavioral_HDL=off  opt=Speed  use_embedded=on  optimum_pipeline=off  pipeline=on  use_rpm=on  placement_style=Triangular  XmcBlockStatus=1  maskContainerNames=group1  block_type=mult  block_config=sysgen:Mult_config  block_width=598  block_height=876
  mult_inp_scale : hdlBasic/Mult  precision=User Defined  arith_type="Signed  (2's comp)"  n_bits=dt.slice.sz  bin_pt=dt.slice.sz - 2  quantization=Truncate  overflow=Wrap  en=off  latency=3  use_behavioral_HDL=off  opt=Speed  use_embedded=on  optimum_pipeline=off  pipeline=on  use_rpm=on  placement_style=Triangular  XmcBlockStatus=1  maskContainerNames=group1  block_type=mult  block_config=sysgen:Mult_config  block_width=598  block_height=876
  mult_out_scale : hdlBasic/Mult  precision=User Defined  arith_type="Signed  (2's comp)"  n_bits=dt.slice.sz  bin_pt=dt.slice.bin  quantization=Truncate  overflow=Wrap  en=off  latency=3  use_behavioral_HDL=off  opt=Speed  use_embedded=on  optimum_pipeline=off  pipeline=on  use_rpm=on  placement_style=Triangular  XmcBlockStatus=1  maskContainerNames=group1  block_type=mult  block_config=sysgen:Mult_config  block_width=598  block_height=876
  reint_sliced : hdlBasic/Reinterpret  force_arith_type=on  arith_type=Unsigned  force_bin_pt=on  bin_pt=dt.slice.bin - ip.f_nlf.lut_addr_bits + 1  XmcBlockStatus=1  maskContainerNames=group1  block_type=reinterpret  block_config=sysgen:Reinterpret_config
  wea_mux : hdlBasic/Mux  inputs=2  en=off  latency=1  precision=Full  arith_type=Unsigned  n_bits=16  bin_pt=14  quantization=Truncate  overflow=Wrap  XmcBlockStatus=1  maskContainerNames=tabcontainer1  block_type=mux  block_config=sysgen:Mux_config
  zero_nlf_datatype : hdlBasic/Constant  const=0  gui_display_data_type=Fixed-point  arith_type=Signed (2's comp)  n_bits=dt.nlf.sz  bin_pt=dt.nlf.bin  preci_type=Single  exp_width=8  frac_width=24  explicit_period=off  period=1  XmcBlockStatus=1  maskContainerNames=tabcontainer1  block_type=constant  block_config=sysgen:Constant_config
  zero_nlf_dina : hdlBasic/Constant  const=0  gui_display_data_type=Fixed-point  arith_type=Signed (2's comp)  n_bits=dt.nlf.sz  bin_pt=dt.nlf.bin  preci_type=Single  exp_width=8  frac_width=24  explicit_period=off  period=1  XmcBlockStatus=1  maskContainerNames=tabcontainer1  block_type=constant  block_config=sysgen:Constant_config
  f(x) : Outport
  wires:
  x/1 -> mult_inp_scale/1
  presc/1 -> mult_inp_scale/2
  cast_cutoff_lsbits/1 -> Reinterpret/1
  Reinterpret/1 -> addra_mux/2, AddSub/1
  const_1/1 -> AddSub/2
  AddSub/1 -> LUT/4
  bool_zero_we/1 -> LUT/6
  zero_nlf_datatype/1 -> LUT/5
  LUT/2 -> mult_b/1
  LUT/1 -> mult_a/1
  mult_inp_scale/1 -> cast_cutoff_lsbits/1, cutoff_msbits/1
  cutoff_msbits/1 -> reint_sliced/1
  reint_sliced/1 -> cast_to_dt/slice/1
  cast_to_dt/slice/1 -> AddSub1/2, delay_sync_interpolate/1
  const_1_interp/1 -> AddSub1/1
  delay_sync_interpolate/1 -> mult_b/2
  AddSub1/1 -> mult_a/2
  mult_a/1 -> add_interpolate/1
  mult_b/1 -> add_interpolate/2
  gain/1 -> mult_out_scale/2
  add_interpolate/1 -> mult_out_scale/1
  mult_out_scale/1 -> f(x)/1
  dina_mux/1 -> LUT/2
  addra_mux/1 -> LUT/1
  wea_mux/1 -> LUT/3
  bool_zero_wea/1 -> wea_mux/2
  zero_nlf_dina/1 -> dina_mux/2
  cfg_select/1 -> wea_mux/1, dina_mux/1, addra_mux/1
  cfg_addr/1 -> addra_mux/3
  cfg_data/1 -> dina_mux/3
  cfg_we/1 -> wea_mux/3
